simulink model "Line_follower_Obj_detect"  (R2022a)
settings: Solver=FixedStepDiscrete  StartTime=0.0  StopTime=10.0  FixedStep=0.1  RelTol=1e-3  EnableMultiTasking=on
undefined symbols (not defined in the file): IR1, IR2
settings Model: Creator=$5CFJ00-M5DIHQERSA94  LastModifiedBy=$5CFJ00-M5DIHQERSA94
settings SolverCC: AlgebraicLoopSolver=TrustRegion  AutoInsertRateTranBlk=on
settings DataIOCC: LimitDataPoints=on
settings OptimizationCC: LifeSpan=inf
settings DebuggingCC: UnconnectedInputMsg=warning  UnconnectedOutputMsg=warning  UnconnectedLineMsg=warning  AllowSymbolicDim=off  SFUnexpectedBacktrackingDiag=warning  SFNoUnconditionalDefaultTransitionDiag=warning  SFExecutionAtInitializationDiag=none  ArithmeticOperatorsInVariantConditions=warning
settings SFSimCC: SimUseLocalCustomCode=off  CustomCodeUndefinedFunction=UseInterfaceOnly
settings RTWCC: RTWUseLocalCustomCode=off  DLArmComputeVersion=19.05
settings CodeAppCC: StateflowObjectComments=on
settings GRTTargetCC: TargetLangStandard=C89/C90 (ANSI)
settings ConfigComp: CovMetricSettings=dw  CovSaveCumulativeToWorkspaceVar=on  CovSaveSingleToWorkspaceVar=on  CovExternalEMLEnable=off  CovSFcnEnable=off

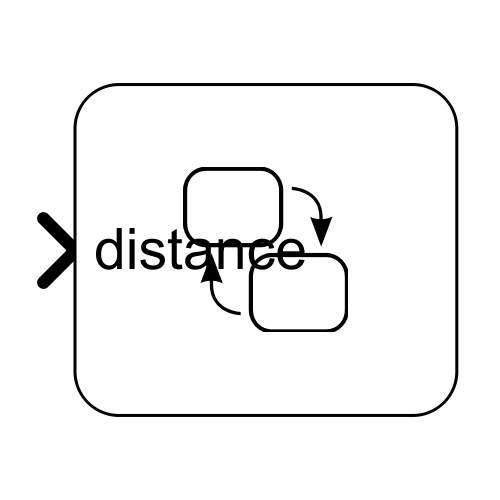
[thumbnail: Simulink's stored preview of the top-level diagram]
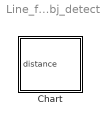
== system Line_follower_Obj_detect ==
  Chart : Stateflow chart  TreatAsAtomicUnit=on

== stateflow chart Line_follower_Obj_detect/Chart ==
  state IR
  state Distance
  state Decider
  state turnRight
  state turnLeft
  state Stop
  state Forward
  (default) -> IR
  Forward -> IR
  turnLeft -> IR
  turnRight -> IR
  IR -> Distance
  Distance -> Decider
  Decider -> turnLeft [order 1] : [IR1 == 0 && IR2 == 1 && distance >= 40]
  Decider -> turnRight [order 4] : [IR1 == 1 && IR2 == 0 && distance >= 40]
  Decider -> Stop [order 3] : [IR1 == 0 && IR2 == 0 &&distance <= 40]
  Decider -> Forward [order 2] : [IR1 == 1 && IR2 == 1 && distance >= 40]
  data: distance input; IR1 parameter; IR2 parameter
